simulink model "example_SQProblem"  (Simulink 8.9)
settings: Solver=VariableStepDiscrete  StartTime=0.0  StopTime=0.5  RelTol=1e-3  EnableMultiTasking=on
undefined symbols (not defined in the file or in its folder): F, H, M2V
settings Model: Creator=jferreau  LastModifiedBy=erich  ExtModeAutoUpdateStatusClock=off
settings OptimizationCC: ExpressionDepthLimit=2147483647  InitFltsAndDblsToZero=on
settings DebuggingCC: SaveWithParameterizedLinksMsg=none  SignalResolutionControl=TryResolveAllWithWarning  SolverPrmCheckMsg=warning
settings GRTTargetCC: TargetFcnLib=ansi_tfl_tmw.mat

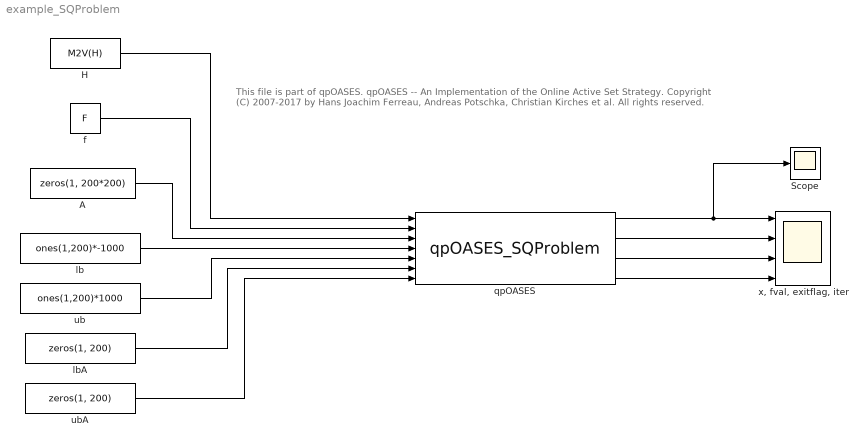
== system example_SQProblem ==
  note: This file is part of qpOASES.
      |
      | qpOASES -- An Implementation of the Online Active Set Strategy.
      | Copyright (C) 2007-2017 by Hans Joachim Ferreau, Andreas Potschka, Christian Kirches et al.
      | All rights reserved.
  A : Constant  Value=zeros(1, 200*200)
  H : Constant  Value=M2V(H)
  Scope : Scope
  f : Constant  Value=F
  lb : Constant  Value=ones(1,200)*-1000
  lbA : Constant  Value=zeros(1, 200)
  qpOASES : S-Function  FunctionName=qpOASES_SQProblem  SFunctionDeploymentMode=off  EnableBusSupport=off
  ub : Constant  Value=ones(1,200)*1000
  ubA : Constant  Value=zeros(1, 200)
  "x, fval, exitflag, iter" : Scope  NumInputPorts=4
  wires:
  qpOASES/1 -> Scope/1, "x, fval, exitflag, iter"/1
  qpOASES/2 -> "x, fval, exitflag, iter"/2
  qpOASES/3 -> "x, fval, exitflag, iter"/3
  qpOASES/4 -> "x, fval, exitflag, iter"/4
  H/1 -> qpOASES/1
  f/1 -> qpOASES/2
  A/1 -> qpOASES/3
  lb/1 -> qpOASES/4
  ub/1 -> qpOASES/5
  lbA/1 -> qpOASES/6
  ubA/1 -> qpOASES/7
